simulink library "ammclib_bam_S32K11x"  (R2016a)
settings: Solver=VariableStepAuto  SolverMode=SingleTasking  StartTime=0.0  StopTime=10.0  RelTol=1e-3
undefined symbols (not defined in the file or in its folder): f16A1, f16A2, f16ADCMaxError, f16B0, f16B1, f16B2, f16C1, f16CC1, f16CC1sc, f16CC1sc_D, f16CC1sc_Q, f16CC2, f16CC2sc, f16CC2sc_D, f16CC2sc_Q, f16DerivGain, f16EGain, f16FiltCoef, f16HystOff, f16HystOn, f16IGain, f16IntegGain, f16IntegGainFW, f16IntegGainQ, f16Kd, f16Kq, f16Limit, f16LowerLimit, f16LowerLimit_D, f16LowerLimit_Q, f16LowerLimitFW, f16LowerLimitQ, f16ModIndex, f16OutValOff, f16OutValOn, f16PropGain, f16PropGainFW, f16PropGainQ, f16RampDown, f16RampUp, f16UGain, f16UpperLimit, f16UpperLimit_D, f16UpperLimit_Q, f16UpperLimitFW, f16UpperLimitQ, f16WIGain, f32A1, f32A2, f32ADCMaxError, f32B0, f32B1, f32B2, f32C1, f32CC1, f32CC1sc, f32CC1sc_D, f32CC1sc_Q, f32CC2, f32CC2sc ... (+62)
(part 11 of 16)

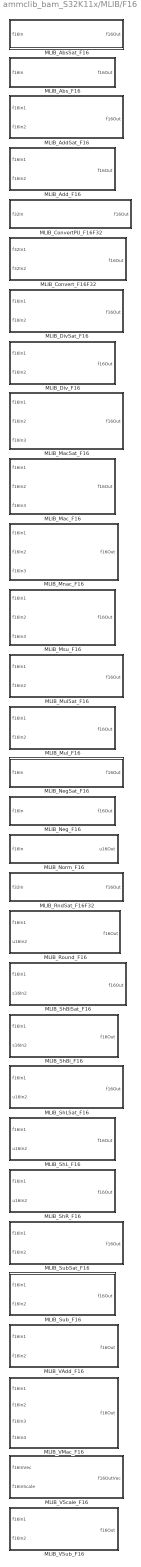
== system ammclib_bam_S32K11x/MLIB/F16 ==
  MLIB_AbsSat_F16 : Subsystem  TreatAsAtomicUnit=on  mask(MLIB_AbsSat_F16){}
      mask help: Saturated absolute value in 16-bit fixed-point fractional implementation. Refer to the AMMCLIB User's Guide for further details.
      mask init: same as ammclib_bam_S32K11x/GDFLIB/F16/GDFLIB_FilterFIR_F16
      settings: RTWSystemCode=Inline
      mask Help: web([fileparts(which('ammclib_bam_S32K11x.slx')) '/../doc/S32K11XMCLUG.pdf'], '-browser')
      mask Display: pos = get_param(gcb, 'Position');width = pos(3) - pos(1); height = pos(4) - pos(2);tX=width/2;tY=height - 8;color('black');text(tX,tY, 'MLIB_AbsSat_F16', 'horizontalAlignment', 'center');
  MLIB_Abs_F16 : Subsystem  TreatAsAtomicUnit=on  mask(MLIB_Abs_F16){}
      mask help: Unsaturated absolute value in 16-bit fixed-point fractional implementation. Refer to the AMMCLIB User's Guide for further details.
      mask init: same as ammclib_bam_S32K11x/GDFLIB/F16/GDFLIB_FilterFIR_F16
      settings: RTWSystemCode=Inline
      mask Help: web([fileparts(which('ammclib_bam_S32K11x.slx')) '/../doc/S32K11XMCLUG.pdf'], '-browser')
      mask Display: pos = get_param(gcb, 'Position');width = pos(3) - pos(1); height = pos(4) - pos(2);tX=width/2;tY=height - 8;color('black');text(tX,tY, 'MLIB_Abs_F16', 'horizontalAlignment', 'center');
  MLIB_AddSat_F16 : Subsystem  TreatAsAtomicUnit=on  mask(MLIB_AddSat_F16){}
      mask help: Saturated addition in 16-bit fixed-point fractional implementation. Refer to the AMMCLIB User's Guide for further details.
      mask init: same as ammclib_bam_S32K11x/GDFLIB/F16/GDFLIB_FilterFIR_F16
      settings: RTWSystemCode=Inline
      mask Help: web([fileparts(which('ammclib_bam_S32K11x.slx')) '/../doc/S32K11XMCLUG.pdf'], '-browser')
      mask Display: pos = get_param(gcb, 'Position');width = pos(3) - pos(1); height = pos(4) - pos(2);tX=width/2;tY=height - 8;color('black');text(tX,tY, 'MLIB_AddSat_F16', 'horizontalAlignment', 'center');
  MLIB_Add_F16 : Subsystem  TreatAsAtomicUnit=on  mask(MLIB_Add_F16){}
      mask help: Unsaturated addition in 16-bit fixed-point fractional implementation.
      mask init: same as ammclib_bam_S32K11x/GDFLIB/F16/GDFLIB_FilterFIR_F16
      settings: RTWSystemCode=Inline
      mask Help: web([fileparts(which('ammclib_bam_S32K11x.slx')) '/../doc/S32K11XMCLUG.pdf'], '-browser')
      mask Display: pos = get_param(gcb, 'Position');width = pos(3) - pos(1); height = pos(4) - pos(2);tX=width/2;tY=height - 8;color('black');text(tX,tY, 'MLIB_Add_F16', 'horizontalAlignment', 'center');
  MLIB_ConvertPU_F16F32 : Subsystem  TreatAsAtomicUnit=on  mask(MLIB_ConvertPU_F16F32){}
      mask help: Conversion of a 32-bit fixed-point fractional value to a 16-bit fixed-point fractional equivalent. Refer to the AMMCLIB User's Guide for further details.
      mask init: same as ammclib_bam_S32K11x/GDFLIB/F16/GDFLIB_FilterFIR_F16
      settings: RTWSystemCode=Inline
      mask Help: web([fileparts(which('ammclib_bam_S32K11x.slx')) '/../doc/S32K11XMCLUG.pdf'], '-browser')
      mask Display: pos = get_param(gcb, 'Position');width = pos(3) - pos(1); height = pos(4) - pos(2);tX=width/2;tY=height - 8;color('black');text(tX,tY, 'MLIB_ConvertPU_F16F32', 'horizontalAlignment', 'center');
  MLIB_Convert_F16F32 : Subsystem  TreatAsAtomicUnit=on  mask(MLIB_Convert_F16F32){}
      mask help: Scaled conversion of a 32-bit fixed-point fractional value to a 16-bit fixed-point fractional equivalent. Refer to the AMMCLIB User's Guide for further details.
      mask init: same as ammclib_bam_S32K11x/GDFLIB/F16/GDFLIB_FilterFIR_F16
      settings: RTWSystemCode=Inline
      mask Help: web([fileparts(which('ammclib_bam_S32K11x.slx')) '/../doc/S32K11XMCLUG.pdf'], '-browser')
      mask Display: pos = get_param(gcb, 'Position');width = pos(3) - pos(1); height = pos(4) - pos(2);tX=width/2;tY=height - 8;color('black');text(tX,tY, 'MLIB_Convert_F16F32', 'horizontalAlignment', 'center');
  MLIB_DivSat_F16 : Subsystem  TreatAsAtomicUnit=on  mask(MLIB_DivSat_F16){}
      mask help: Saturated division of two input values in 16-bit fixed-point fractional implementation. Refer to the AMMCLIB User's Guide for further details.
      mask init: same as ammclib_bam_S32K11x/GDFLIB/F16/GDFLIB_FilterFIR_F16
      settings: RTWSystemCode=Inline
      mask Help: web([fileparts(which('ammclib_bam_S32K11x.slx')) '/../doc/S32K11XMCLUG.pdf'], '-browser')
      mask Display: pos = get_param(gcb, 'Position');width = pos(3) - pos(1); height = pos(4) - pos(2);tX=width/2;tY=height - 8;color('black');text(tX,tY, 'MLIB_DivSat_F16', 'horizontalAlignment', 'center');
  MLIB_Div_F16 : Subsystem  TreatAsAtomicUnit=on  mask(MLIB_Div_F16){}
      mask help: Division of two input values without saturation in 16-bit fixed-point fractional implementation. Refer to the AMMCLIB User's Guide for further details.
      mask init: same as ammclib_bam_S32K11x/GDFLIB/F16/GDFLIB_FilterFIR_F16
      settings: RTWSystemCode=Inline
      mask Help: web([fileparts(which('ammclib_bam_S32K11x.slx')) '/../doc/S32K11XMCLUG.pdf'], '-browser')
      mask Display: pos = get_param(gcb, 'Position');width = pos(3) - pos(1); height = pos(4) - pos(2);tX=width/2;tY=height - 8;color('black');text(tX,tY, 'MLIB_Div_F16', 'horizontalAlignment', 'center');
  MLIB_MacSat_F16 : Subsystem  TreatAsAtomicUnit=on  mask(MLIB_MacSat_F16){}
      mask help: Saturated multiply-accumulate of input values in 16-bit fixed-point fractional implementation. Refer to the AMMCLIB User's Guide for further details.
      mask init: same as ammclib_bam_S32K11x/GDFLIB/F16/GDFLIB_FilterFIR_F16
      settings: RTWSystemCode=Inline
      mask Help: web([fileparts(which('ammclib_bam_S32K11x.slx')) '/../doc/S32K11XMCLUG.pdf'], '-browser')
      mask Display: pos = get_param(gcb, 'Position');width = pos(3) - pos(1); height = pos(4) - pos(2);tX=width/2;tY=height - 8;color('black');text(tX,tY, 'MLIB_MacSat_F16', 'horizontalAlignment', 'center');
  MLIB_Mac_F16 : Subsystem  TreatAsAtomicUnit=on  mask(MLIB_Mac_F16){}
      mask help: Unsaturated multiply-accumulate function in 16-bit fixed-point fractional implementation. Refer to the AMMCLIB User's Guide for further details.
      mask init: same as ammclib_bam_S32K11x/GDFLIB/F16/GDFLIB_FilterFIR_F16
      settings: RTWSystemCode=Inline
      mask Help: web([fileparts(which('ammclib_bam_S32K11x.slx')) '/../doc/S32K11XMCLUG.pdf'], '-browser')
      mask Display: pos = get_param(gcb, 'Position');width = pos(3) - pos(1); height = pos(4) - pos(2);tX=width/2;tY=height - 8;color('black');text(tX,tY, 'MLIB_Mac_F16', 'horizontalAlignment', 'center');
  MLIB_Mnac_F16 : Subsystem  TreatAsAtomicUnit=on  mask(MLIB_Mnac_F16){}
      mask help: Unsaturated multiply-negative-accumulate function in 16-bit fixed-point fractional implementation. Refer to the AMMCLIB User's Guide for further details.
      mask init: same as ammclib_bam_S32K11x/GDFLIB/F16/GDFLIB_FilterFIR_F16
      settings: RTWSystemCode=Inline
      mask Help: web([fileparts(which('ammclib_bam_S32K11x.slx')) '/../doc/S32K11XMCLUG.pdf'], '-browser')
      mask Display: pos = get_param(gcb, 'Position');width = pos(3) - pos(1); height = pos(4) - pos(2);tX=width/2;tY=height - 8;color('black');text(tX,tY, 'MLIB_Mnac_F16', 'horizontalAlignment', 'center');
  MLIB_Msu_F16 : Subsystem  TreatAsAtomicUnit=on  mask(MLIB_Msu_F16){}
      mask help: Unsaturated multiply-subtract-from function in 16-bit fixed-point fractional implementation. Refer to the AMMCLIB User's Guide for further details.
      mask init: same as ammclib_bam_S32K11x/GDFLIB/F16/GDFLIB_FilterFIR_F16
      settings: RTWSystemCode=Inline
      mask Help: web([fileparts(which('ammclib_bam_S32K11x.slx')) '/../doc/S32K11XMCLUG.pdf'], '-browser')
      mask Display: pos = get_param(gcb, 'Position');width = pos(3) - pos(1); height = pos(4) - pos(2);tX=width/2;tY=height - 8;color('black');text(tX,tY, 'MLIB_Msu_F16', 'horizontalAlignment', 'center');
  MLIB_MulSat_F16 : Subsystem  TreatAsAtomicUnit=on  mask(MLIB_MulSat_F16){}
      mask help: Saturated multiplication of two input values in 16-bit fixed-point fractional implementation. Refer to the AMMCLIB User's Guide for further details.
      mask init: same as ammclib_bam_S32K11x/GDFLIB/F16/GDFLIB_FilterFIR_F16
      settings: RTWSystemCode=Inline
      mask Help: web([fileparts(which('ammclib_bam_S32K11x.slx')) '/../doc/S32K11XMCLUG.pdf'], '-browser')
      mask Display: pos = get_param(gcb, 'Position');width = pos(3) - pos(1); height = pos(4) - pos(2);tX=width/2;tY=height - 8;color('black');text(tX,tY, 'MLIB_MulSat_F16', 'horizontalAlignment', 'center');
  MLIB_Mul_F16 : Subsystem  TreatAsAtomicUnit=on  mask(MLIB_Mul_F16){}
      mask help: Unsaturated multiplication of two input values in 16-bit fixed-point fractional implementation. Refer to the AMMCLIB User's Guide for further details.
      mask init: same as ammclib_bam_S32K11x/GDFLIB/F16/GDFLIB_FilterFIR_F16
      settings: RTWSystemCode=Inline
      mask Help: web([fileparts(which('ammclib_bam_S32K11x.slx')) '/../doc/S32K11XMCLUG.pdf'], '-browser')
      mask Display: pos = get_param(gcb, 'Position');width = pos(3) - pos(1); height = pos(4) - pos(2);tX=width/2;tY=height - 8;color('black');text(tX,tY, 'MLIB_Mul_F16', 'horizontalAlignment', 'center');
  MLIB_NegSat_F16 : Subsystem  TreatAsAtomicUnit=on  mask(MLIB_NegSat_F16){}
      mask help: Saturated negation in 16-bit fixed-point fractional implementation. Refer to the AMMCLIB User's Guide for further details.
      mask init: same as ammclib_bam_S32K11x/GDFLIB/F16/GDFLIB_FilterFIR_F16
      settings: RTWSystemCode=Inline
      mask Help: web([fileparts(which('ammclib_bam_S32K11x.slx')) '/../doc/S32K11XMCLUG.pdf'], '-browser')
      mask Display: pos = get_param(gcb, 'Position');width = pos(3) - pos(1); height = pos(4) - pos(2);tX=width/2;tY=height - 8;color('black');text(tX,tY, 'MLIB_NegSat_F16', 'horizontalAlignment', 'center');
  MLIB_Neg_F16 : Subsystem  TreatAsAtomicUnit=on  mask(MLIB_Neg_F16){}
      mask help: Unsaturated negation in 16-bit fixed-point fractional implementation. Refer to the AMMCLIB User's Guide for further details.
      mask init: same as ammclib_bam_S32K11x/GDFLIB/F16/GDFLIB_FilterFIR_F16
      settings: RTWSystemCode=Inline
      mask Help: web([fileparts(which('ammclib_bam_S32K11x.slx')) '/../doc/S32K11XMCLUG.pdf'], '-browser')
      mask Display: pos = get_param(gcb, 'Position');width = pos(3) - pos(1); height = pos(4) - pos(2);tX=width/2;tY=height - 8;color('black');text(tX,tY, 'MLIB_Neg_F16', 'horizontalAlignment', 'center');
  MLIB_Norm_F16 : Subsystem  TreatAsAtomicUnit=on  mask(MLIB_Norm_F16){}
      mask help: Normalization function in 16-bit fixed-point fractional implementation. The function counts the number of left shift needed for normalization of the input fractional value. Refer to the AMMCLIB User's Guide for further details.
      mask init: same as ammclib_bam_S32K11x/GDFLIB/F16/GDFLIB_FilterFIR_F16
      settings: RTWSystemCode=Inline
      mask Help: web([fileparts(which('ammclib_bam_S32K11x.slx')) '/../doc/S32K11XMCLUG.pdf'], '-browser')
      mask Display: pos = get_param(gcb, 'Position');width = pos(3) - pos(1); height = pos(4) - pos(2);tX=width/2;tY=height - 8;color('black');text(tX,tY, 'MLIB_Norm_F16', 'horizontalAlignment', 'center');
  MLIB_RndSat_F16F32 : Subsystem  TreatAsAtomicUnit=on  mask(MLIB_RndSat_F16F32){}
      mask help: Saturated round to the nearest 16-bit fractional value. Refer to the AMMCLIB User's Guide for further details.
      mask init: same as ammclib_bam_S32K11x/GDFLIB/F16/GDFLIB_FilterFIR_F16
      settings: RTWSystemCode=Inline
      mask Help: web([fileparts(which('ammclib_bam_S32K11x.slx')) '/../doc/S32K11XMCLUG.pdf'], '-browser')
      mask Display: pos = get_param(gcb, 'Position');width = pos(3) - pos(1); height = pos(4) - pos(2);tX=width/2;tY=height - 8;color('black');text(tX,tY, 'MLIB_RndSat_F16F32', 'horizontalAlignment', 'center');
  MLIB_Round_F16 : Subsystem  TreatAsAtomicUnit=on  mask(MLIB_Round_F16){}
      mask help: Rounding function in 16-bit fixed-point fractional implementation. The function rounds the first input value to the number of digits defined by second input value and saturates the result. Refer to the AMMCLIB User's Guide for further details.
      mask init: same as ammclib_bam_S32K11x/GDFLIB/F16/GDFLIB_FilterFIR_F16
      settings: RTWSystemCode=Inline
      mask Help: web([fileparts(which('ammclib_bam_S32K11x.slx')) '/../doc/S32K11XMCLUG.pdf'], '-browser')
      mask Display: pos = get_param(gcb, 'Position');width = pos(3) - pos(1); height = pos(4) - pos(2);tX=width/2;tY=height - 8;color('black');text(tX,tY, 'MLIB_Round_F16', 'horizontalAlignment', 'center');
  MLIB_ShBiSat_F16 : Subsystem  TreatAsAtomicUnit=on  mask(MLIB_ShBiSat_F16){}
      mask help: Saturated bidirectional shift in 16-bit fixed-point fractional implementation. The function shifts the first input value to the left (if the second input is negative) or right (if the second input is positive) by the amount defined by second input value, saturating the result. Refer to the AMMCLIB User's Guide for further details.
      mask init: same as ammclib_bam_S32K11x/GDFLIB/F16/GDFLIB_FilterFIR_F16
      settings: RTWSystemCode=Inline
      mask Help: web([fileparts(which('ammclib_bam_S32K11x.slx')) '/../doc/S32K11XMCLUG.pdf'], '-browser')
      mask Display: pos = get_param(gcb, 'Position');width = pos(3) - pos(1); height = pos(4) - pos(2);tX=width/2;tY=height - 8;color('black');text(tX,tY, 'MLIB_ShBiSat_F16', 'horizontalAlignment', 'center');
  MLIB_ShBi_F16 : Subsystem  TreatAsAtomicUnit=on  mask(MLIB_ShBi_F16){}
      mask help: Unsaturated bidirectional shift in 16-bit fixed-point fractional implementation. The function shifts the first input value to the left (if the second input is negative) or right (if the second input is positive) by the amount defined by second input value. Refer to the AMMCLIB User's Guide for further details.
      mask init: same as ammclib_bam_S32K11x/GDFLIB/F16/GDFLIB_FilterFIR_F16
      settings: RTWSystemCode=Inline
      mask Help: web([fileparts(which('ammclib_bam_S32K11x.slx')) '/../doc/S32K11XMCLUG.pdf'], '-browser')
      mask Display: pos = get_param(gcb, 'Position');width = pos(3) - pos(1); height = pos(4) - pos(2);tX=width/2;tY=height - 8;color('black');text(tX,tY, 'MLIB_ShBi_F16', 'horizontalAlignment', 'center');
  MLIB_ShLSat_F16 : Subsystem  TreatAsAtomicUnit=on  mask(MLIB_ShLSat_F16){}
      mask help: Saturated shift left in 16-bit fixed-point fractional implementation. The function shifts the first input value to the left by the amount defined by the second input value, saturating the result. Refer to the AMMCLIB User's Guide for further details.
      mask init: same as ammclib_bam_S32K11x/GDFLIB/F16/GDFLIB_FilterFIR_F16
      settings: RTWSystemCode=Inline
      mask Help: web([fileparts(which('ammclib_bam_S32K11x.slx')) '/../doc/S32K11XMCLUG.pdf'], '-browser')
      mask Display: pos = get_param(gcb, 'Position');width = pos(3) - pos(1); height = pos(4) - pos(2);tX=width/2;tY=height - 8;color('black');text(tX,tY, 'MLIB_ShLSat_F16', 'horizontalAlignment', 'center');
  MLIB_ShL_F16 : Subsystem  TreatAsAtomicUnit=on  mask(MLIB_ShL_F16){}
      mask help: Unsaturated shift left in 16-bit fixed-point fractional implementation. The function shifts the first input value to the left by the amount defined by the second input value. Refer to the AMMCLIB User's Guide for further details.
      mask init: same as ammclib_bam_S32K11x/GDFLIB/F16/GDFLIB_FilterFIR_F16
      settings: RTWSystemCode=Inline
      mask Help: web([fileparts(which('ammclib_bam_S32K11x.slx')) '/../doc/S32K11XMCLUG.pdf'], '-browser')
      mask Display: pos = get_param(gcb, 'Position');width = pos(3) - pos(1); height = pos(4) - pos(2);tX=width/2;tY=height - 8;color('black');text(tX,tY, 'MLIB_ShL_F16', 'horizontalAlignment', 'center');
  MLIB_ShR_F16 : Subsystem  TreatAsAtomicUnit=on  mask(MLIB_ShR_F16){}
      mask help: Unsaturated shift right in 16-bit fixed-point fractional implementation. The function shifts the first input value to the right by the amount defined by the second input value. Refer to the AMMCLIB User's Guide for further details.
      mask init: same as ammclib_bam_S32K11x/GDFLIB/F16/GDFLIB_FilterFIR_F16
      settings: RTWSystemCode=Inline
      mask Help: web([fileparts(which('ammclib_bam_S32K11x.slx')) '/../doc/S32K11XMCLUG.pdf'], '-browser')
      mask Display: pos = get_param(gcb, 'Position');width = pos(3) - pos(1); height = pos(4) - pos(2);tX=width/2;tY=height - 8;color('black');text(tX,tY, 'MLIB_ShR_F16', 'horizontalAlignment', 'center');
  MLIB_SubSat_F16 : Subsystem  TreatAsAtomicUnit=on  mask(MLIB_SubSat_F16){}
      mask help: Saturated subtraction in 16-bit fixed-point fractional implementation. Refer to the AMMCLIB User's Guide for further details.
      mask init: same as ammclib_bam_S32K11x/GDFLIB/F16/GDFLIB_FilterFIR_F16
      settings: RTWSystemCode=Inline
      mask Help: web([fileparts(which('ammclib_bam_S32K11x.slx')) '/../doc/S32K11XMCLUG.pdf'], '-browser')
      mask Display: pos = get_param(gcb, 'Position');width = pos(3) - pos(1); height = pos(4) - pos(2);tX=width/2;tY=height - 8;color('black');text(tX,tY, 'MLIB_SubSat_F16', 'horizontalAlignment', 'center');
  MLIB_Sub_F16 : Subsystem  TreatAsAtomicUnit=on  mask(MLIB_Sub_F16){}
      mask help: Unsaturated subtraction in 16-bit fixed-point fractional implementation. Refer to the AMMCLIB User's Guide for further details.
      mask init: same as ammclib_bam_S32K11x/GDFLIB/F16/GDFLIB_FilterFIR_F16
      settings: RTWSystemCode=Inline
      mask Help: web([fileparts(which('ammclib_bam_S32K11x.slx')) '/../doc/S32K11XMCLUG.pdf'], '-browser')
      mask Display: pos = get_param(gcb, 'Position');width = pos(3) - pos(1); height = pos(4) - pos(2);tX=width/2;tY=height - 8;color('black');text(tX,tY, 'MLIB_Sub_F16', 'horizontalAlignment', 'center');
  MLIB_VAdd_F16 : Subsystem  TreatAsAtomicUnit=on  mask(MLIB_VAdd_F16){}
      mask help: Vector addition in 16-bit fixed-point fractional implementation.
      mask init: same as ammclib_bam_S32K11x/GDFLIB/F16/GDFLIB_FilterFIR_F16
      settings: RTWSystemCode=Inline
      mask Help: web([fileparts(which('ammclib_bam_S32K11x.slx')) '/../doc/S32K11XMCLUG.pdf'], '-browser')
      mask Display: pos = get_param(gcb, 'Position');width = pos(3) - pos(1); height = pos(4) - pos(2);tX=width/2;tY=height - 8;color('black');text(tX,tY, 'MLIB_VAdd_F16', 'horizontalAlignment', 'center');
  MLIB_VMac_F16 : Subsystem  TreatAsAtomicUnit=on  mask(MLIB_VMac_F16){}
      mask help: Dot product of 2-element vectors with saturated multiplication and modulo accumulation in 16-bit fixed-point fractional implementation. Refer to the AMMCLIB User's Guide for further details.
      mask init: same as ammclib_bam_S32K11x/GDFLIB/F16/GDFLIB_FilterFIR_F16
      settings: RTWSystemCode=Inline
      mask Help: web([fileparts(which('ammclib_bam_S32K11x.slx')) '/../doc/S32K11XMCLUG.pdf'], '-browser')
      mask Display: pos = get_param(gcb, 'Position');width = pos(3) - pos(1); height = pos(4) - pos(2);tX=width/2;tY=height - 8;color('black');text(tX,tY, 'MLIB_VMac_F16', 'horizontalAlignment', 'center');
  MLIB_VScale_F16 : Subsystem  TreatAsAtomicUnit=on  mask(MLIB_VScale_F16){}
      mask help: Multiplication of a vector and scalar in 16-bit fixed-point fractional implementation.
      mask init: same as ammclib_bam_S32K11x/GDFLIB/F16/GDFLIB_FilterFIR_F16
      settings: RTWSystemCode=Inline
      mask Help: web([fileparts(which('ammclib_bam_S32K11x.slx')) '/../doc/S32K11XMCLUG.pdf'], '-browser')
      mask Display: pos = get_param(gcb, 'Position');width = pos(3) - pos(1); height = pos(4) - pos(2);tX=width/2;tY=height - 8;color('black');text(tX,tY, 'MLIB_VScale_F16', 'horizontalAlignment', 'center');
  MLIB_VSub_F16 : Subsystem  TreatAsAtomicUnit=on  mask(MLIB_VSub_F16){}
      mask help: Vector substraction in 16-bit fixed-point fractional implementation.
      mask init: same as ammclib_bam_S32K11x/GDFLIB/F16/GDFLIB_FilterFIR_F16
      settings: RTWSystemCode=Inline
      mask Help: web([fileparts(which('ammclib_bam_S32K11x.slx')) '/../doc/S32K11XMCLUG.pdf'], '-browser')
      mask Display: pos = get_param(gcb, 'Position');width = pos(3) - pos(1); height = pos(4) - pos(2);tX=width/2;tY=height - 8;color('black');text(tX,tY, 'MLIB_VSub_F16', 'horizontalAlignment', 'center');

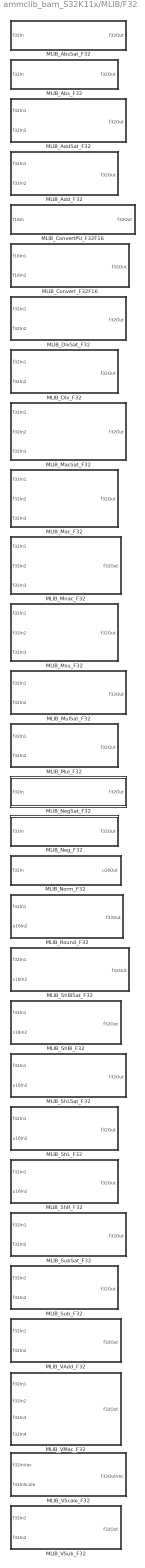
== system ammclib_bam_S32K11x/MLIB/F32 ==
  MLIB_AbsSat_F32 : Subsystem  TreatAsAtomicUnit=on  mask(MLIB_AbsSat_F32){}
      mask help: Saturated absolute value in 32-bit fixed-point fractional implementation. Refer to the AMMCLIB User's Guide for further details.
      mask init: same as ammclib_bam_S32K11x/GDFLIB/F16/GDFLIB_FilterFIR_F16
      settings: RTWSystemCode=Inline
      mask Help: web([fileparts(which('ammclib_bam_S32K11x.slx')) '/../doc/S32K11XMCLUG.pdf'], '-browser')
      mask Display: pos = get_param(gcb, 'Position');width = pos(3) - pos(1); height = pos(4) - pos(2);tX=width/2;tY=height - 8;color('black');text(tX,tY, 'MLIB_AbsSat_F32', 'horizontalAlignment', 'center');
  MLIB_Abs_F32 : Subsystem  TreatAsAtomicUnit=on  mask(MLIB_Abs_F32){}
      mask help: Unsaturated absolute value in 32-bit fixed-point fractional implementation. Refer to the AMMCLIB User's Guide for further details.
      mask init: same as ammclib_bam_S32K11x/GDFLIB/F16/GDFLIB_FilterFIR_F16
      settings: RTWSystemCode=Inline
      mask Help: web([fileparts(which('ammclib_bam_S32K11x.slx')) '/../doc/S32K11XMCLUG.pdf'], '-browser')
      mask Display: pos = get_param(gcb, 'Position');width = pos(3) - pos(1); height = pos(4) - pos(2);tX=width/2;tY=height - 8;color('black');text(tX,tY, 'MLIB_Abs_F32', 'horizontalAlignment', 'center');
  MLIB_AddSat_F32 : Subsystem  TreatAsAtomicUnit=on  mask(MLIB_AddSat_F32){}
      mask help: Saturated addition in 32-bit fixed-point fractional implementation. Refer to the AMMCLIB User's Guide for further details.
      mask init: same as ammclib_bam_S32K11x/GDFLIB/F16/GDFLIB_FilterFIR_F16
      settings: RTWSystemCode=Inline
      mask Help: web([fileparts(which('ammclib_bam_S32K11x.slx')) '/../doc/S32K11XMCLUG.pdf'], '-browser')
      mask Display: pos = get_param(gcb, 'Position');width = pos(3) - pos(1); height = pos(4) - pos(2);tX=width/2;tY=height - 8;color('black');text(tX,tY, 'MLIB_AddSat_F32', 'horizontalAlignment', 'center');
  MLIB_Add_F32 : Subsystem  TreatAsAtomicUnit=on  mask(MLIB_Add_F32){}
      mask help: Unsaturated addition in 32-bit fixed-point fractional implementation.
      mask init: same as ammclib_bam_S32K11x/GDFLIB/F16/GDFLIB_FilterFIR_F16
      settings: RTWSystemCode=Inline
      mask Help: web([fileparts(which('ammclib_bam_S32K11x.slx')) '/../doc/S32K11XMCLUG.pdf'], '-browser')
      mask Display: pos = get_param(gcb, 'Position');width = pos(3) - pos(1); height = pos(4) - pos(2);tX=width/2;tY=height - 8;color('black');text(tX,tY, 'MLIB_Add_F32', 'horizontalAlignment', 'center');
  MLIB_ConvertPU_F32F16 : Subsystem  TreatAsAtomicUnit=on  mask(MLIB_ConvertPU_F32F16){}
      mask help: Conversion of a 16-bit fixed-point fractional value to a 32-bit fixed-point fractional equivalent. Refer to the AMMCLIB User's Guide for further details.
      mask init: same as ammclib_bam_S32K11x/GDFLIB/F16/GDFLIB_FilterFIR_F16
      settings: RTWSystemCode=Inline
      mask Help: web([fileparts(which('ammclib_bam_S32K11x.slx')) '/../doc/S32K11XMCLUG.pdf'], '-browser')
      mask Display: pos = get_param(gcb, 'Position');width = pos(3) - pos(1); height = pos(4) - pos(2);tX=width/2;tY=height - 8;color('black');text(tX,tY, 'MLIB_ConvertPU_F32F16', 'horizontalAlignment', 'center');
  MLIB_Convert_F32F16 : Subsystem  TreatAsAtomicUnit=on  mask(MLIB_Convert_F32F16){}
      mask help: Scaled conversion of a 16-bit fixed-point fractional value to a 32-bit fixed-point fractional equivalent. Refer to the AMMCLIB User's Guide for further details.
      mask init: same as ammclib_bam_S32K11x/GDFLIB/F16/GDFLIB_FilterFIR_F16
      settings: RTWSystemCode=Inline
      mask Help: web([fileparts(which('ammclib_bam_S32K11x.slx')) '/../doc/S32K11XMCLUG.pdf'], '-browser')
      mask Display: pos = get_param(gcb, 'Position');width = pos(3) - pos(1); height = pos(4) - pos(2);tX=width/2;tY=height - 8;color('black');text(tX,tY, 'MLIB_Convert_F32F16', 'horizontalAlignment', 'center');
  MLIB_DivSat_F32 : Subsystem  TreatAsAtomicUnit=on  mask(MLIB_DivSat_F32){}
      mask help: Saturated division of two input values in 32-bit fixed-point fractional implementation. Refer to the AMMCLIB User's Guide for further details.
      mask init: same as ammclib_bam_S32K11x/GDFLIB/F16/GDFLIB_FilterFIR_F16
      settings: RTWSystemCode=Inline
      mask Help: web([fileparts(which('ammclib_bam_S32K11x.slx')) '/../doc/S32K11XMCLUG.pdf'], '-browser')
      mask Display: pos = get_param(gcb, 'Position');width = pos(3) - pos(1); height = pos(4) - pos(2);tX=width/2;tY=height - 8;color('black');text(tX,tY, 'MLIB_DivSat_F32', 'horizontalAlignment', 'center');
  MLIB_Div_F32 : Subsystem  TreatAsAtomicUnit=on  mask(MLIB_Div_F32){}
      mask help: Division of two input values without saturation in 32-bit fixed-point fractional implementation. Refer to the AMMCLIB User's Guide for further details.
      mask init: same as ammclib_bam_S32K11x/GDFLIB/F16/GDFLIB_FilterFIR_F16
      settings: RTWSystemCode=Inline
      mask Help: web([fileparts(which('ammclib_bam_S32K11x.slx')) '/../doc/S32K11XMCLUG.pdf'], '-browser')
      mask Display: pos = get_param(gcb, 'Position');width = pos(3) - pos(1); height = pos(4) - pos(2);tX=width/2;tY=height - 8;color('black');text(tX,tY, 'MLIB_Div_F32', 'horizontalAlignment', 'center');
  MLIB_MacSat_F32 : Subsystem  TreatAsAtomicUnit=on  mask(MLIB_MacSat_F32){}
      mask help: Saturated multiply-accumulate of input values in 32-bit fixed-point fractional implementation. Refer to the AMMCLIB User's Guide for further details.
      mask init: same as ammclib_bam_S32K11x/GDFLIB/F16/GDFLIB_FilterFIR_F16
      settings: RTWSystemCode=Inline
      mask Help: web([fileparts(which('ammclib_bam_S32K11x.slx')) '/../doc/S32K11XMCLUG.pdf'], '-browser')
      mask Display: pos = get_param(gcb, 'Position');width = pos(3) - pos(1); height = pos(4) - pos(2);tX=width/2;tY=height - 8;color('black');text(tX,tY, 'MLIB_MacSat_F32', 'horizontalAlignment', 'center');
  MLIB_Mac_F32 : Subsystem  TreatAsAtomicUnit=on  mask(MLIB_Mac_F32){}
      mask help: Unsaturated multiply-accumulate function in 32-bit fixed-point fractional implementation. Refer to the AMMCLIB User's Guide for further details.
      mask init: same as ammclib_bam_S32K11x/GDFLIB/F16/GDFLIB_FilterFIR_F16
      settings: RTWSystemCode=Inline
      mask Help: web([fileparts(which('ammclib_bam_S32K11x.slx')) '/../doc/S32K11XMCLUG.pdf'], '-browser')
      mask Display: pos = get_param(gcb, 'Position');width = pos(3) - pos(1); height = pos(4) - pos(2);tX=width/2;tY=height - 8;color('black');text(tX,tY, 'MLIB_Mac_F32', 'horizontalAlignment', 'center');
  MLIB_Mnac_F32 : Subsystem  TreatAsAtomicUnit=on  mask(MLIB_Mnac_F32){}
      mask help: Unsaturated multiply-negative-accumulate function in 32-bit fixed-point fractional implementation. Refer to the AMMCLIB User's Guide for further details.
      mask init: same as ammclib_bam_S32K11x/GDFLIB/F16/GDFLIB_FilterFIR_F16
      settings: RTWSystemCode=Inline
      mask Help: web([fileparts(which('ammclib_bam_S32K11x.slx')) '/../doc/S32K11XMCLUG.pdf'], '-browser')
      mask Display: pos = get_param(gcb, 'Position');width = pos(3) - pos(1); height = pos(4) - pos(2);tX=width/2;tY=height - 8;color('black');text(tX,tY, 'MLIB_Mnac_F32', 'horizontalAlignment', 'center');
  MLIB_Msu_F32 : Subsystem  TreatAsAtomicUnit=on  mask(MLIB_Msu_F32){}
      mask help: Unsaturated multiply-subtract-from function in 32-bit fixed-point fractional implementation. Refer to the AMMCLIB User's Guide for further details.
      mask init: same as ammclib_bam_S32K11x/GDFLIB/F16/GDFLIB_FilterFIR_F16
      settings: RTWSystemCode=Inline
      mask Help: web([fileparts(which('ammclib_bam_S32K11x.slx')) '/../doc/S32K11XMCLUG.pdf'], '-browser')
      mask Display: pos = get_param(gcb, 'Position');width = pos(3) - pos(1); height = pos(4) - pos(2);tX=width/2;tY=height - 8;color('black');text(tX,tY, 'MLIB_Msu_F32', 'horizontalAlignment', 'center');
  MLIB_MulSat_F32 : Subsystem  TreatAsAtomicUnit=on  mask(MLIB_MulSat_F32){}
      mask help: Saturated multiplication of two input values in 32-bit fixed-point fractional implementation. Refer to the AMMCLIB User's Guide for further details.
      mask init: same as ammclib_bam_S32K11x/GDFLIB/F16/GDFLIB_FilterFIR_F16
      settings: RTWSystemCode=Inline
      mask Help: web([fileparts(which('ammclib_bam_S32K11x.slx')) '/../doc/S32K11XMCLUG.pdf'], '-browser')
      mask Display: pos = get_param(gcb, 'Position');width = pos(3) - pos(1); height = pos(4) - pos(2);tX=width/2;tY=height - 8;color('black');text(tX,tY, 'MLIB_MulSat_F32', 'horizontalAlignment', 'center');
  MLIB_Mul_F32 : Subsystem  TreatAsAtomicUnit=on  mask(MLIB_Mul_F32){}
      mask help: Unsaturated multiplication of two input values in 32-bit fixed-point fractional implementation. Refer to the AMMCLIB User's Guide for further details.
      mask init: same as ammclib_bam_S32K11x/GDFLIB/F16/GDFLIB_FilterFIR_F16
      settings: RTWSystemCode=Inline
      mask Help: web([fileparts(which('ammclib_bam_S32K11x.slx')) '/../doc/S32K11XMCLUG.pdf'], '-browser')
      mask Display: pos = get_param(gcb, 'Position');width = pos(3) - pos(1); height = pos(4) - pos(2);tX=width/2;tY=height - 8;color('black');text(tX,tY, 'MLIB_Mul_F32', 'horizontalAlignment', 'center');
  MLIB_NegSat_F32 : Subsystem  TreatAsAtomicUnit=on  mask(MLIB_NegSat_F32){}
      mask help: Saturated negation in 32-bit fixed-point fractional implementation. Refer to the AMMCLIB User's Guide for further details.
      mask init: same as ammclib_bam_S32K11x/GDFLIB/F16/GDFLIB_FilterFIR_F16
      settings: RTWSystemCode=Inline
      mask Help: web([fileparts(which('ammclib_bam_S32K11x.slx')) '/../doc/S32K11XMCLUG.pdf'], '-browser')
      mask Display: pos = get_param(gcb, 'Position');width = pos(3) - pos(1); height = pos(4) - pos(2);tX=width/2;tY=height - 8;color('black');text(tX,tY, 'MLIB_NegSat_F32', 'horizontalAlignment', 'center');
  MLIB_Neg_F32 : Subsystem  TreatAsAtomicUnit=on  mask(MLIB_Neg_F32){}
      mask help: Unsaturated negation in 32-bit fixed-point fractional implementation. Refer to the AMMCLIB User's Guide for further details.
      mask init: same as ammclib_bam_S32K11x/GDFLIB/F16/GDFLIB_FilterFIR_F16
      settings: RTWSystemCode=Inline
      mask Help: web([fileparts(which('ammclib_bam_S32K11x.slx')) '/../doc/S32K11XMCLUG.pdf'], '-browser')
      mask Display: pos = get_param(gcb, 'Position');width = pos(3) - pos(1); height = pos(4) - pos(2);tX=width/2;tY=height - 8;color('black');text(tX,tY, 'MLIB_Neg_F32', 'horizontalAlignment', 'center');
  MLIB_Norm_F32 : Subsystem  TreatAsAtomicUnit=on  mask(MLIB_Norm_F32){}
      mask help: Normalization function in 32-bit fixed-point fractional implementation. The function counts the number of left shift needed for normalization of the input fractional value. Refer to the AMMCLIB User's Guide for further details.
      mask init: same as ammclib_bam_S32K11x/GDFLIB/F16/GDFLIB_FilterFIR_F16
      settings: RTWSystemCode=Inline
      mask Help: web([fileparts(which('ammclib_bam_S32K11x.slx')) '/../doc/S32K11XMCLUG.pdf'], '-browser')
      mask Display: pos = get_param(gcb, 'Position');width = pos(3) - pos(1); height = pos(4) - pos(2);tX=width/2;tY=height - 8;color('black');text(tX,tY, 'MLIB_Norm_F32', 'horizontalAlignment', 'center');
  MLIB_Round_F32 : Subsystem  TreatAsAtomicUnit=on  mask(MLIB_Round_F32){}
      mask help: Rounding function in 32-bit fixed-point fractional implementation. The function rounds the first input value to the number of digits defined by second input value and saturates the result. Refer to the AMMCLIB User's Guide for further details.
      mask init: same as ammclib_bam_S32K11x/GDFLIB/F16/GDFLIB_FilterFIR_F16
      settings: RTWSystemCode=Inline
      mask Help: web([fileparts(which('ammclib_bam_S32K11x.slx')) '/../doc/S32K11XMCLUG.pdf'], '-browser')
      mask Display: pos = get_param(gcb, 'Position');width = pos(3) - pos(1); height = pos(4) - pos(2);tX=width/2;tY=height - 8;color('black');text(tX,tY, 'MLIB_Round_F32', 'horizontalAlignment', 'center');
  MLIB_ShBiSat_F32 : Subsystem  TreatAsAtomicUnit=on  mask(MLIB_ShBiSat_F32){}
      mask help: Saturated bidirectional shift in 32-bit fixed-point fractional implementation. The function shifts the first input value to the left (if the second input is negative) or right (if the second input is positive) by the amount defined by second input value, saturating the result. Refer to the AMMCLIB User's Guide for further details.
      mask init: same as ammclib_bam_S32K11x/GDFLIB/F16/GDFLIB_FilterFIR_F16
      settings: RTWSystemCode=Inline
      mask Help: web([fileparts(which('ammclib_bam_S32K11x.slx')) '/../doc/S32K11XMCLUG.pdf'], '-browser')
      mask Display: pos = get_param(gcb, 'Position');width = pos(3) - pos(1); height = pos(4) - pos(2);tX=width/2;tY=height - 8;color('black');text(tX,tY, 'MLIB_ShBiSat_F32', 'horizontalAlignment', 'center');
  MLIB_ShBi_F32 : Subsystem  TreatAsAtomicUnit=on  mask(MLIB_ShBi_F32){}
      mask help: Unsaturated bidirectional shift in 32-bit fixed-point fractional implementation. The function shifts the first input value to the left (if the second input is negative) or right (if the second input is positive) by the amount defined by second input value. Refer to the AMMCLIB User's Guide for further details.
      mask init: same as ammclib_bam_S32K11x/GDFLIB/F16/GDFLIB_FilterFIR_F16
      settings: RTWSystemCode=Inline
      mask Help: web([fileparts(which('ammclib_bam_S32K11x.slx')) '/../doc/S32K11XMCLUG.pdf'], '-browser')
      mask Display: pos = get_param(gcb, 'Position');width = pos(3) - pos(1); height = pos(4) - pos(2);tX=width/2;tY=height - 8;color('black');text(tX,tY, 'MLIB_ShBi_F32', 'horizontalAlignment', 'center');
  MLIB_ShLSat_F32 : Subsystem  TreatAsAtomicUnit=on  mask(MLIB_ShLSat_F32){}
      mask help: Saturated shift left in 32-bit fixed-point fractional implementation. The function shifts the first input value to the left by the amount defined by the second input value, saturating the result. Refer to the AMMCLIB User's Guide for further details.
      mask init: same as ammclib_bam_S32K11x/GDFLIB/F16/GDFLIB_FilterFIR_F16
      settings: RTWSystemCode=Inline
      mask Help: web([fileparts(which('ammclib_bam_S32K11x.slx')) '/../doc/S32K11XMCLUG.pdf'], '-browser')
      mask Display: pos = get_param(gcb, 'Position');width = pos(3) - pos(1); height = pos(4) - pos(2);tX=width/2;tY=height - 8;color('black');text(tX,tY, 'MLIB_ShLSat_F32', 'horizontalAlignment', 'center');
  MLIB_ShL_F32 : Subsystem  TreatAsAtomicUnit=on  mask(MLIB_ShL_F32){}
      mask help: Unsaturated shift left in 32-bit fixed-point fractional implementation. The function shifts the first input value to the left by the amount defined by the second input value. Refer to the AMMCLIB User's Guide for further details.
      mask init: same as ammclib_bam_S32K11x/GDFLIB/F16/GDFLIB_FilterFIR_F16
      settings: RTWSystemCode=Inline
      mask Help: web([fileparts(which('ammclib_bam_S32K11x.slx')) '/../doc/S32K11XMCLUG.pdf'], '-browser')
      mask Display: pos = get_param(gcb, 'Position');width = pos(3) - pos(1); height = pos(4) - pos(2);tX=width/2;tY=height - 8;color('black');text(tX,tY, 'MLIB_ShL_F32', 'horizontalAlignment', 'center');
  MLIB_ShR_F32 : Subsystem  TreatAsAtomicUnit=on  mask(MLIB_ShR_F32){}
      mask help: Unsaturated shift right in 32-bit fixed-point fractional implementation. The function shifts the first input value to the right by the amount defined by the second input value. Refer to the AMMCLIB User's Guide for further details.
      mask init: same as ammclib_bam_S32K11x/GDFLIB/F16/GDFLIB_FilterFIR_F16
      settings: RTWSystemCode=Inline
      mask Help: web([fileparts(which('ammclib_bam_S32K11x.slx')) '/../doc/S32K11XMCLUG.pdf'], '-browser')
      mask Display: pos = get_param(gcb, 'Position');width = pos(3) - pos(1); height = pos(4) - pos(2);tX=width/2;tY=height - 8;color('black');text(tX,tY, 'MLIB_ShR_F32', 'horizontalAlignment', 'center');
  MLIB_SubSat_F32 : Subsystem  TreatAsAtomicUnit=on  mask(MLIB_SubSat_F32){}
      mask help: Saturated subtraction in 32-bit fixed-point fractional implementation. Refer to the AMMCLIB User's Guide for further details.
      mask init: same as ammclib_bam_S32K11x/GDFLIB/F16/GDFLIB_FilterFIR_F16
      settings: RTWSystemCode=Inline
      mask Help: web([fileparts(which('ammclib_bam_S32K11x.slx')) '/../doc/S32K11XMCLUG.pdf'], '-browser')
      mask Display: pos = get_param(gcb, 'Position');width = pos(3) - pos(1); height = pos(4) - pos(2);tX=width/2;tY=height - 8;color('black');text(tX,tY, 'MLIB_SubSat_F32', 'horizontalAlignment', 'center');
  MLIB_Sub_F32 : Subsystem  TreatAsAtomicUnit=on  mask(MLIB_Sub_F32){}
      mask help: Unsaturated subtraction in 32-bit fixed-point fractional implementation. Refer to the AMMCLIB User's Guide for further details.
      mask init: same as ammclib_bam_S32K11x/GDFLIB/F16/GDFLIB_FilterFIR_F16
      settings: RTWSystemCode=Inline
      mask Help: web([fileparts(which('ammclib_bam_S32K11x.slx')) '/../doc/S32K11XMCLUG.pdf'], '-browser')
      mask Display: pos = get_param(gcb, 'Position');width = pos(3) - pos(1); height = pos(4) - pos(2);tX=width/2;tY=height - 8;color('black');text(tX,tY, 'MLIB_Sub_F32', 'horizontalAlignment', 'center');
  MLIB_VAdd_F32 : Subsystem  TreatAsAtomicUnit=on  mask(MLIB_VAdd_F32){}
      mask help: Vector addition in 32-bit fixed-point fractional implementation.
      mask init: same as ammclib_bam_S32K11x/GDFLIB/F16/GDFLIB_FilterFIR_F16
      settings: RTWSystemCode=Inline
      mask Help: web([fileparts(which('ammclib_bam_S32K11x.slx')) '/../doc/S32K11XMCLUG.pdf'], '-browser')
      mask Display: pos = get_param(gcb, 'Position');width = pos(3) - pos(1); height = pos(4) - pos(2);tX=width/2;tY=height - 8;color('black');text(tX,tY, 'MLIB_VAdd_F32', 'horizontalAlignment', 'center');
  MLIB_VMac_F32 : Subsystem  TreatAsAtomicUnit=on  mask(MLIB_VMac_F32){}
      mask help: Dot product of 2-element vectors with saturated multiplication and modulo accumulation in 32-bit fixed-point fractional implementation. Refer to the AMMCLIB User's Guide for further details.
      mask init: same as ammclib_bam_S32K11x/GDFLIB/F16/GDFLIB_FilterFIR_F16
      settings: RTWSystemCode=Inline
      mask Help: web([fileparts(which('ammclib_bam_S32K11x.slx')) '/../doc/S32K11XMCLUG.pdf'], '-browser')
      mask Display: pos = get_param(gcb, 'Position');width = pos(3) - pos(1); height = pos(4) - pos(2);tX=width/2;tY=height - 8;color('black');text(tX,tY, 'MLIB_VMac_F32', 'horizontalAlignment', 'center');
  MLIB_VScale_F32 : Subsystem  TreatAsAtomicUnit=on  mask(MLIB_VScale_F32){}
      mask help: Multiplication of a vector and scalar in 32-bit fixed-point fractional implementation.
      mask init: same as ammclib_bam_S32K11x/GDFLIB/F16/GDFLIB_FilterFIR_F16
      settings: RTWSystemCode=Inline
      mask Help: web([fileparts(which('ammclib_bam_S32K11x.slx')) '/../doc/S32K11XMCLUG.pdf'], '-browser')
      mask Display: pos = get_param(gcb, 'Position');width = pos(3) - pos(1); height = pos(4) - pos(2);tX=width/2;tY=height - 8;color('black');text(tX,tY, 'MLIB_VScale_F32', 'horizontalAlignment', 'center');
  MLIB_VSub_F32 : Subsystem  TreatAsAtomicUnit=on  mask(MLIB_VSub_F32){}
      mask help: Vector substraction in 32-bit fixed-point fractional implementation.
      mask init: same as ammclib_bam_S32K11x/GDFLIB/F16/GDFLIB_FilterFIR_F16
      settings: RTWSystemCode=Inline
      mask Help: web([fileparts(which('ammclib_bam_S32K11x.slx')) '/../doc/S32K11XMCLUG.pdf'], '-browser')
      mask Display: pos = get_param(gcb, 'Position');width = pos(3) - pos(1); height = pos(4) - pos(2);tX=width/2;tY=height - 8;color('black');text(tX,tY, 'MLIB_VSub_F32', 'horizontalAlignment', 'center');

== system ammclib_bam_S32K11x/MLIB/F32F16F16 ==
  MLIB_MacSat_F32F16F16 : Subsystem  TreatAsAtomicUnit=on  mask(MLIB_MacSat_F32F16F16){}
      mask help: Saturated multiply-accumulate of input values in 16/32-bit fixed-point fractional implementation. Refer to the AMMCLIB User's Guide for further details.
      mask init: same as ammclib_bam_S32K11x/GDFLIB/F16/GDFLIB_FilterFIR_F16
      settings: RTWSystemCode=Inline
      mask Help: web([fileparts(which('ammclib_bam_S32K11x.slx')) '/../doc/S32K11XMCLUG.pdf'], '-browser')
      mask Display: pos = get_param(gcb, 'Position');width = pos(3) - pos(1); height = pos(4) - pos(2);tX=width/2;tY=height - 8;color('black');text(tX,tY, 'MLIB_MacSat_F32F16F16', 'horizontalAlignment', 'center');
  MLIB_Mac_F32F16F16 : Subsystem  TreatAsAtomicUnit=on  mask(MLIB_Mac_F32F16F16){}
      mask help: Unsaturated multiply-accumulate function in 16/32-bit fixed-point fractional implementation. Refer to the AMMCLIB User's Guide for further details.
      mask init: same as ammclib_bam_S32K11x/GDFLIB/F16/GDFLIB_FilterFIR_F16
      settings: RTWSystemCode=Inline
      mask Help: web([fileparts(which('ammclib_bam_S32K11x.slx')) '/../doc/S32K11XMCLUG.pdf'], '-browser')
      mask Display: pos = get_param(gcb, 'Position');width = pos(3) - pos(1); height = pos(4) - pos(2);tX=width/2;tY=height - 8;color('black');text(tX,tY, 'MLIB_Mac_F32F16F16', 'horizontalAlignment', 'center');
  MLIB_Mnac_F32F16F16 : Subsystem  TreatAsAtomicUnit=on  mask(MLIB_Mnac_F32F16F16){}
      mask help: Unsaturated multiply-negative-accumulate function in 16/32-bit fixed-point fractional implementation. Refer to the AMMCLIB User's Guide for further details.
      mask init: same as ammclib_bam_S32K11x/GDFLIB/F16/GDFLIB_FilterFIR_F16
      settings: RTWSystemCode=Inline
      mask Help: web([fileparts(which('ammclib_bam_S32K11x.slx')) '/../doc/S32K11XMCLUG.pdf'], '-browser')
      mask Display: pos = get_param(gcb, 'Position');width = pos(3) - pos(1); height = pos(4) - pos(2);tX=width/2;tY=height - 8;color('black');text(tX,tY, 'MLIB_Mnac_F32F16F16', 'horizontalAlignment', 'center');
  MLIB_Msu_F32F16F16 : Subsystem  TreatAsAtomicUnit=on  mask(MLIB_Msu_F32F16F16){}
      mask help: Unsaturated multiply-subtract-from function in 16/32-bit fixed-point fractional implementation. Refer to the AMMCLIB User's Guide for further details.
      mask init: same as ammclib_bam_S32K11x/GDFLIB/F16/GDFLIB_FilterFIR_F16
      settings: RTWSystemCode=Inline
      mask Help: web([fileparts(which('ammclib_bam_S32K11x.slx')) '/../doc/S32K11XMCLUG.pdf'], '-browser')
      mask Display: pos = get_param(gcb, 'Position');width = pos(3) - pos(1); height = pos(4) - pos(2);tX=width/2;tY=height - 8;color('black');text(tX,tY, 'MLIB_Msu_F32F16F16', 'horizontalAlignment', 'center');
  MLIB_MulSat_F32F16F16 : Subsystem  TreatAsAtomicUnit=on  mask(MLIB_MulSat_F32F16F16){}
      mask help: Saturated multiplication of two input values in 16/32-bit fixed-point fractional implementation. Refer to the AMMCLIB User's Guide for further details.
      mask init: same as ammclib_bam_S32K11x/GDFLIB/F16/GDFLIB_FilterFIR_F16
      settings: RTWSystemCode=Inline
      mask Help: web([fileparts(which('ammclib_bam_S32K11x.slx')) '/../doc/S32K11XMCLUG.pdf'], '-browser')
      mask Display: pos = get_param(gcb, 'Position');width = pos(3) - pos(1); height = pos(4) - pos(2);tX=width/2;tY=height - 8;color('black');text(tX,tY, 'MLIB_MulSat_F32F16F16', 'horizontalAlignment', 'center');
  MLIB_Mul_F32F16F16 : Subsystem  TreatAsAtomicUnit=on  mask(MLIB_Mul_F32F16F16){}
      mask help: Unsaturated multiplication of two input values in 16/32-bit fixed-point fractional implementation. Refer to the AMMCLIB User's Guide for further details.
      mask init: same as ammclib_bam_S32K11x/GDFLIB/F16/GDFLIB_FilterFIR_F16
      settings: RTWSystemCode=Inline
      mask Help: web([fileparts(which('ammclib_bam_S32K11x.slx')) '/../doc/S32K11XMCLUG.pdf'], '-browser')
      mask Display: pos = get_param(gcb, 'Position');width = pos(3) - pos(1); height = pos(4) - pos(2);tX=width/2;tY=height - 8;color('black');text(tX,tY, 'MLIB_Mul_F32F16F16', 'horizontalAlignment', 'center');
  MLIB_VMac_F32F16F16 : Subsystem  TreatAsAtomicUnit=on  mask(MLIB_VMac_F32F16F16){}
      mask help: Dot product of 2-element vectors with saturated multiplication and modulo accumulation in 16/32-bit fixed-point fractional implementation. Refer to the AMMCLIB User's Guide for further details.
      mask init: same as ammclib_bam_S32K11x/GDFLIB/F16/GDFLIB_FilterFIR_F16
      settings: RTWSystemCode=Inline
      mask Help: web([fileparts(which('ammclib_bam_S32K11x.slx')) '/../doc/S32K11XMCLUG.pdf'], '-browser')
      mask Display: pos = get_param(gcb, 'Position');width = pos(3) - pos(1); height = pos(4) - pos(2);tX=width/2;tY=height - 8;color('black');text(tX,tY, 'MLIB_VMac_F32F16F16', 'horizontalAlignment', 'center');

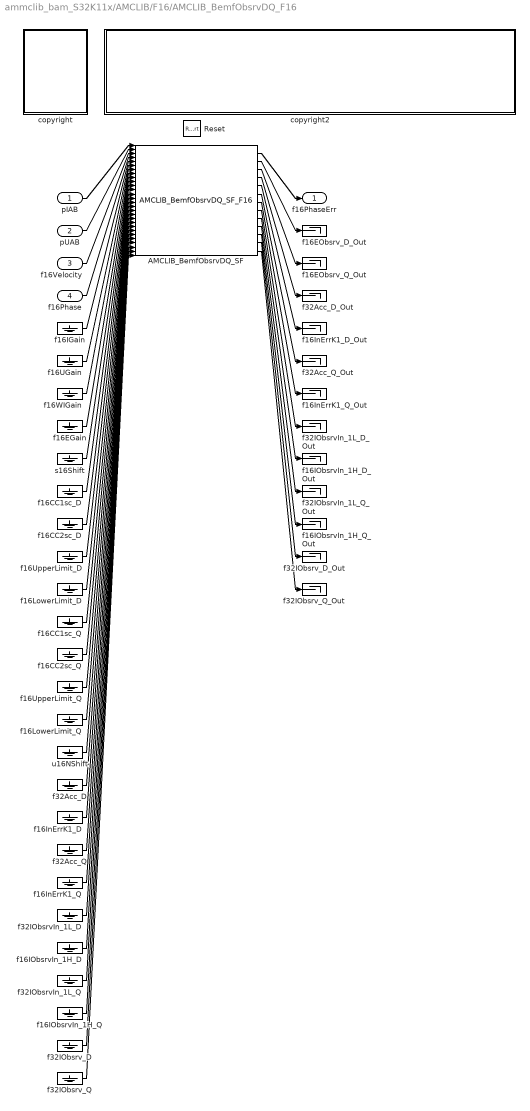
== system ammclib_bam_S32K11x/AMCLIB/F16/AMCLIB_BemfObsrvDQ_F16 ==
  pIAB : Inport  OutDataTypeStr=Bus: SWLIBS_2Syst_F16  BusOutputAsStruct=on
  pUAB : Inport  Port=2  OutDataTypeStr=Bus: SWLIBS_2Syst_F16  BusOutputAsStruct=on
  f16Velocity : Inport  Port=3  OutDataTypeStr=int16
  f16Phase : Inport  Port=4  OutDataTypeStr=int16
  Reset : ResetPort  DisableCoverage=on
  AMCLIB_BemfObsrvDQ_SF : S-Function  FunctionName=AMCLIB_BemfObsrvDQ_SF_F16  Parameters=showStates,resetStatesEnable,f16IGain,f16UGain,f16WIGain,f16EGain,s16Shift,f16CC1sc_D,f16CC2sc_D,f16UpperLimit_D,f16LowerLimit_D,f16CC1sc_Q,f16CC2sc_Q,f16UpperLimit_Q,f16LowerLimit_Q,u16NShift  SFunctionDeploymentMode=off  EnableBusSupport=off
  copyright : Subsystem
      mask Display: text(10,90,'FILE:');text(10,75,'DESRIPTION:');text(10,60,'COPYRIGHT:');text(10,45,'VERSION:');text(10,30,'DATE:')
  copyright2 : Subsystem
      mask Display: text(10,90,'AMCLIB_BemfObsrvDQ_BAM_F16.mdl');text(10,75,'PMSM back-EMF observer DQ.');text(10,60,'NXP 2020');text(10,45,'1.0');text(10,30,'28-Mar-2020');
  f16CC1sc_D : Ground
  f16CC1sc_Q : Ground
  f16CC2sc_D : Ground
  f16CC2sc_Q : Ground
  f16EGain : Ground
  f16EObsrv_D_Out : Terminator
  f16EObsrv_Q_Out : Terminator
  f16IGain : Ground
  f16IObsrvIn_1H_D : Ground
  f16IObsrvIn_1H_D_Out : Terminator
  f16IObsrvIn_1H_Q : Ground
  f16IObsrvIn_1H_Q_Out : Terminator
  f16InErrK1_D : Ground
  f16InErrK1_D_Out : Terminator
  f16InErrK1_Q : Ground
  f16InErrK1_Q_Out : Terminator
  f16LowerLimit_D : Ground
  f16LowerLimit_Q : Ground
  f16UGain : Ground
  f16UpperLimit_D : Ground
  f16UpperLimit_Q : Ground
  f16WIGain : Ground
  f32Acc_D : Ground
  f32Acc_D_Out : Terminator
  f32Acc_Q : Ground
  f32Acc_Q_Out : Terminator
  f32IObsrvIn_1L_D : Ground
  f32IObsrvIn_1L_D_Out : Terminator
  f32IObsrvIn_1L_Q : Ground
  f32IObsrvIn_1L_Q_Out : Terminator
  f32IObsrv_D : Ground
  f32IObsrv_D_Out : Terminator
  f32IObsrv_Q : Ground
  f32IObsrv_Q_Out : Terminator
  s16Shift : Ground
  u16NShift : Ground
  f16PhaseErr : Outport
  wires:
  AMCLIB_BemfObsrvDQ_SF/13 -> f32IObsrv_Q_Out/1
  AMCLIB_BemfObsrvDQ_SF/12 -> f32IObsrv_D_Out/1
  AMCLIB_BemfObsrvDQ_SF/11 -> f16IObsrvIn_1H_Q_Out/1
  AMCLIB_BemfObsrvDQ_SF/10 -> f32IObsrvIn_1L_Q_Out/1
  AMCLIB_BemfObsrvDQ_SF/9 -> f16IObsrvIn_1H_D_Out/1
  AMCLIB_BemfObsrvDQ_SF/8 -> f32IObsrvIn_1L_D_Out/1
  AMCLIB_BemfObsrvDQ_SF/7 -> f16InErrK1_Q_Out/1
  AMCLIB_BemfObsrvDQ_SF/6 -> f32Acc_Q_Out/1
  AMCLIB_BemfObsrvDQ_SF/5 -> f16InErrK1_D_Out/1
  AMCLIB_BemfObsrvDQ_SF/4 -> f32Acc_D_Out/1
  AMCLIB_BemfObsrvDQ_SF/3 -> f16EObsrv_Q_Out/1
  AMCLIB_BemfObsrvDQ_SF/2 -> f16EObsrv_D_Out/1
  AMCLIB_BemfObsrvDQ_SF/1 -> f16PhaseErr/1
  f32IObsrv_Q/1 -> AMCLIB_BemfObsrvDQ_SF/28
  f32IObsrv_D/1 -> AMCLIB_BemfObsrvDQ_SF/27
  f16IObsrvIn_1H_Q/1 -> AMCLIB_BemfObsrvDQ_SF/26
  f32IObsrvIn_1L_Q/1 -> AMCLIB_BemfObsrvDQ_SF/25
  f16IObsrvIn_1H_D/1 -> AMCLIB_BemfObsrvDQ_SF/24
  f32IObsrvIn_1L_D/1 -> AMCLIB_BemfObsrvDQ_SF/23
  f16InErrK1_Q/1 -> AMCLIB_BemfObsrvDQ_SF/22
  f32Acc_Q/1 -> AMCLIB_BemfObsrvDQ_SF/21
  f16InErrK1_D/1 -> AMCLIB_BemfObsrvDQ_SF/20
  f32Acc_D/1 -> AMCLIB_BemfObsrvDQ_SF/19
  u16NShift/1 -> AMCLIB_BemfObsrvDQ_SF/18
  f16LowerLimit_Q/1 -> AMCLIB_BemfObsrvDQ_SF/17
  f16UpperLimit_Q/1 -> AMCLIB_BemfObsrvDQ_SF/16
  f16CC2sc_Q/1 -> AMCLIB_BemfObsrvDQ_SF/15
  f16CC1sc_Q/1 -> AMCLIB_BemfObsrvDQ_SF/14
  f16LowerLimit_D/1 -> AMCLIB_BemfObsrvDQ_SF/13
  f16UpperLimit_D/1 -> AMCLIB_BemfObsrvDQ_SF/12
  f16CC2sc_D/1 -> AMCLIB_BemfObsrvDQ_SF/11
  f16CC1sc_D/1 -> AMCLIB_BemfObsrvDQ_SF/10
  s16Shift/1 -> AMCLIB_BemfObsrvDQ_SF/9
  f16EGain/1 -> AMCLIB_BemfObsrvDQ_SF/8
  f16WIGain/1 -> AMCLIB_BemfObsrvDQ_SF/7
  f16UGain/1 -> AMCLIB_BemfObsrvDQ_SF/6
  f16IGain/1 -> AMCLIB_BemfObsrvDQ_SF/5
  f16Phase/1 -> AMCLIB_BemfObsrvDQ_SF/4
  f16Velocity/1 -> AMCLIB_BemfObsrvDQ_SF/3
  pUAB/1 -> AMCLIB_BemfObsrvDQ_SF/2
  pIAB/1 -> AMCLIB_BemfObsrvDQ_SF/1
